simulink model "VariableMotorWiringPi"  (R2015a)
settings: Solver=ode3  StartTime=0.0  StopTime=0.5  FixedStep=0.0001  RelTol=1e-3
settings Model: SimulationMode=external  ExtModeTrigDuration=100  Creator=Justin  LastModifiedBy=Justin
settings OptimizationCC: OptimizeModelRefInitCode=on  LifeSpan=1
settings DebuggingCC: ParameterOverflowMsg=warning
settings HardwareCC: ProdLargestAtomicInteger=Long  ProdLargestAtomicFloat=Double  ProdEndianess=LittleEndian  ProdHWDeviceType=ARM Compatible->ARM Cortex
settings RTWCC: SystemTargetFile=realtime.tlc  GenerateMakefile=off  TemplateMakefile=realtime.tmf  Description=Run on Target Hardware  RTWVerbose=off
settings ERTTargetCC: CombineOutputUpdateFcns=off  ERTSrcFileBannerTemplate=realtime_code_template.cgt  ERTHdrFileBannerTemplate=realtime_code_template.cgt  ERTDataSrcFileTemplate=realtime_code_template.cgt  ERTDataHdrFileTemplate=realtime_code_template.cgt  ERTCustomFileTemplate=realtime_file_process.tlc

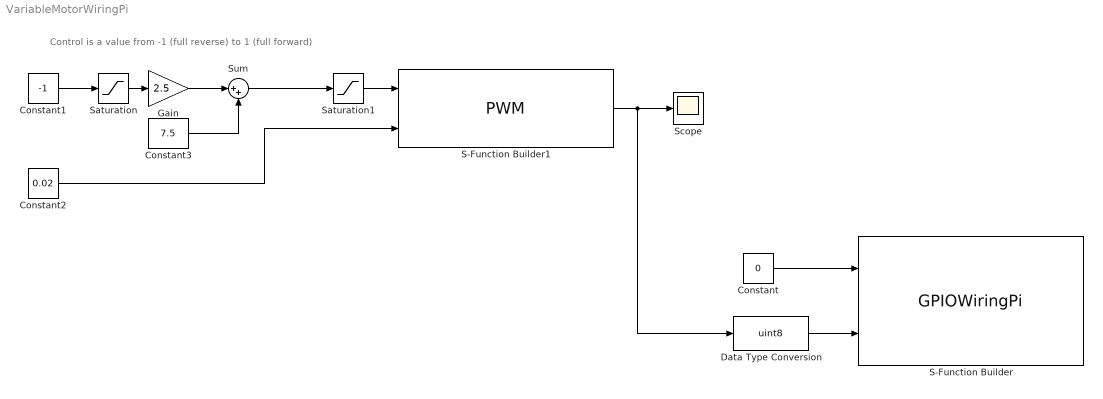
== system VariableMotorWiringPi ==
  note: Control is a value from -1 (full reverse) to 1 (full forward)
  Constant : Constant  Value=0  OutDataTypeStr=uint8
  Constant1 : Constant  Value=-1  OutDataTypeStr=uint8
  Constant2 : Constant  Value=0.02
  Constant3 : Constant  Value=7.5
  Data Type Conversion : DataTypeConversion  OutDataTypeStr=uint8
  Gain : Gain  Gain=2.5
  S-Function Builder : S-Function  InitFcn=try, set_param(gcb,'FunctionName','GPIOWiringPi'), end  FunctionName=GPIOWiringPi  SFunctionModules=GPIOWiringPi_wrapper  mask(S-Function Builder){}
      mask help: Simulink:masks:SFunctionBuilder_MD
      mask init:
      | val = [[.9  0.75 0.75 1 1 .9 .9 1]',[1 1 0.75 0.75 .9 .9 1 .9]'];try , sys = get_param(gcb,'SfunBuilderFcnName');if isempty(sys), sys = get_param(gcb,'FunctionName'); end,catch, sys = get_param(gcb,'FunctionName'); end
      settings: CopyFcn=set_param(gcbh,'LinkStatus','none')  PreSaveFcn=try, set_param(gcb,'FunctionName','GPIOWiringPi'), end  OpenFcn=sfunctionwizard(gcbh)
      mask Display: plot(val(:,1),val(:,2)),disp(sys), port_label('input',1,'GPIO_Number'), port_label('input',2,'GPIO_Value')
  S-Function Builder1 : S-Function  InitFcn=try, set_param(gcb,'FunctionName','PWM'), end  FunctionName=PWM  SFunctionModules=PWM_wrapper  mask(S-Function Builder){}
      mask help: Simulink:masks:SFunctionBuilder_MD
      mask init: same as VariableMotorWiringPi/S-Function Builder
      settings: CopyFcn=set_param(gcbh,'LinkStatus','none')  PreSaveFcn=try, set_param(gcb,'FunctionName','PWM'), end  OpenFcn=sfunctionwizard(gcbh)
      mask Display:
      | plot(val(:,1),val(:,2))
      | disp(sys)
      | port_label('input',1,'PulseWidth')
      | port_label('input',2,'Period')
      | port_label('output',1,'SignalOutput')
  Saturation : Saturate  UpperLimit=1  LowerLimit=-1
  Saturation1 : Saturate  UpperLimit=100  LowerLimit=0.1
  Scope : Scope
  Sum : Sum  Inputs=|++
  wires:
  Sum/1 -> Saturation1/1
  Saturation1/1 -> S-Function Builder1/1
  Constant2/1 -> S-Function Builder1/2
  Constant1/1 -> Saturation/1
  Saturation/1 -> Gain/1
  Gain/1 -> Sum/1
  Constant3/1 -> Sum/2
  Constant/1 -> S-Function Builder/1
  S-Function Builder1/1 -> Data Type Conversion/1, Scope/1
  Data Type Conversion/1 -> S-Function Builder/2
